simulink model "arduino_controller"  (R2019b)
settings: Solver=VariableStepAuto  StartTime=0.0  StopTime=500  RelTol=1e-3  EnableMultiTasking=on
StartFcn:
  | clear all
undefined symbols (not defined in the file or in its folder): A, B, C, D, Tnom_celsius
libraries: realtime_pacer_lib x1
settings Model: Creator=johnh  LastModifiedBy=Presentatie
settings DataIOCC: ReturnWorkspaceOutputs=off
settings OptimizationCC: LifeSpan=inf
settings DebuggingCC: SFUnexpectedBacktrackingDiag=warning  SFNoUnconditionalDefaultTransitionDiag=warning  SFExecutionAtInitializationDiag=none  ArithmeticOperatorsInVariantConditions=warning
settings SFSimCC: SimUseLocalCustomCode=off  CustomCodeUndefinedFunction=UseInterfaceOnly
settings RTWCC: RTWUseLocalCustomCode=off
settings CodeAppCC: StateflowObjectComments=on
settings GRTTargetCC: TargetLangStandard=C89/C90 (ANSI)  GeneratePreprocessorConditionals=Disable all
settings ConfigComp: CovMetricSettings=dw  CovHtmlReporting=on  CovSaveCumulativeToWorkspaceVar=on  CovSaveSingleToWorkspaceVar=on  CovExternalEMLEnable=off

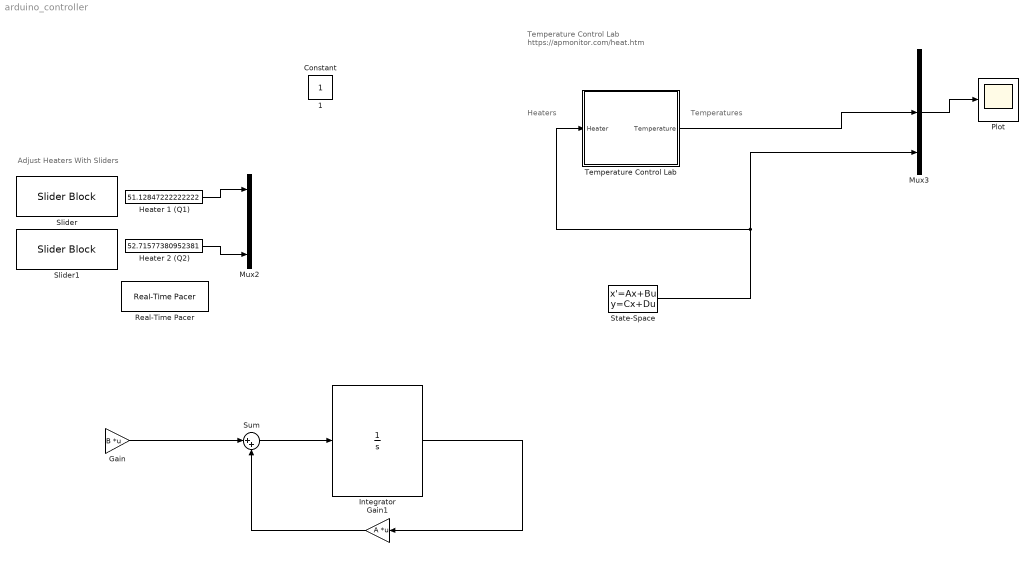
== system arduino_controller ==
  note: Adjust Heaters With Sliders
  note: Temperature Control Lab
      | https://apmonitor.com/heat.htm
  note: Heaters
  note: Temperatures
  Gain : Gain  Gain=B  Multiplication=Matrix(K*u)
  Gain1 : Gain  Gain=A  Multiplication=Matrix(K*u)
  Heater 1 (Q1) : Constant  Value=51.12847222222222
  Heater 2 (Q2) : Constant  Value=52.71577380952381
  Integrator : Integrator  InitialCondition=Tnom_celsius
  Mux2 : Mux  Inputs=3
  Mux3 : Mux  Inputs=3
  Plot : Scope
  Real-Time Pacer : realtime_pacer_lib/Real-Time Pacer  simTimePerRealTime=1
  Slider : SliderBlock  TickInterval=20
  Slider1 : SliderBlock  TickInterval=20
  State-Space : StateSpace  A=A  B=B  C=C  D=D  InitialCondition=Tnom_celsius  ContinuousStateAttributes="\"\""
  Sum : Sum  Inputs=|++
  Temperature Control Lab : Subsystem
      mask Display: image('tclab.png');
  1 : Constant  IOType=siggen
  Constant : Constant  IOType=siggen
  wires:
  Heater 1 (Q1)/1 -> Mux2/1
  Heater 2 (Q2)/1 -> Mux2/3
  Mux3/1 -> Plot/1
  State-Space/1 -> Temperature Control Lab/1(Heater), Mux3/3
  Temperature Control Lab/1(Temperature) -> Mux3/2
  Integrator/1 -> Gain1/1
  Sum/1 -> Integrator/1
  Gain1/1 -> Sum/2
  Gain/1 -> Sum/1

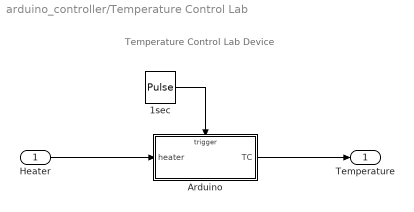
== system arduino_controller/Temperature Control Lab ==
  note: Temperature Control Lab Device
  Heater : Inport
  1sec : DiscretePulseGenerator  PulseType=Time based  Period=1  PulseWidth=50
  Arduino : Subsystem  TreatAsAtomicUnit=on
  Temperature : Outport  VectorParamsAs1DForOutWhenUnconnected=off
  wires:
  1sec/1 -> Arduino/Trigger
  Arduino/1(TC) -> Temperature/1
  Heater/1 -> Arduino/1(heater)

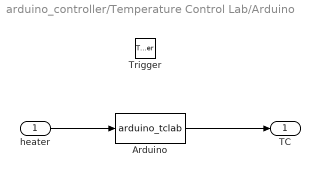
== system arduino_controller/Temperature Control Lab/Arduino ==
  heater : Inport  LatchByDelayingOutsideSignal=on
  Trigger : TriggerPort  VariantControl=Variant
  Arduino : MATLABFcn  MATLABFcn=arduino_tclab
  TC : Outport  InitialOutput=[23 23]  VectorParamsAs1DForOutWhenUnconnected=off
  wires:
  heater/1 -> Arduino/1
  Arduino/1 -> TC/1
